simulink model "lab1"  (R2022a)
settings: Solver=FixedStepAuto  StartTime=0.0  StopTime=1e6  RelTol=1e-3
InitFcn:
  | lab1
settings Model: Creator=Natriya  LastModifiedBy=Natriya

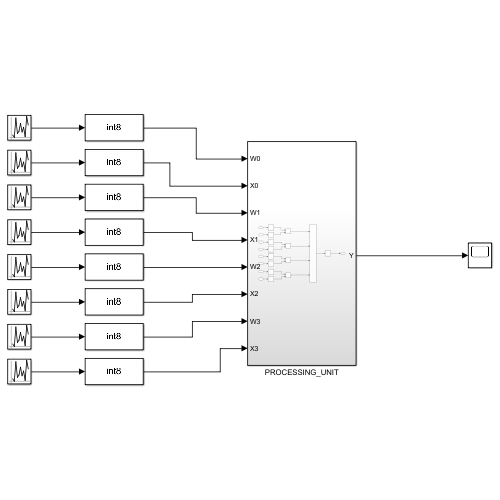
[thumbnail: Simulink's stored preview of the top-level diagram]
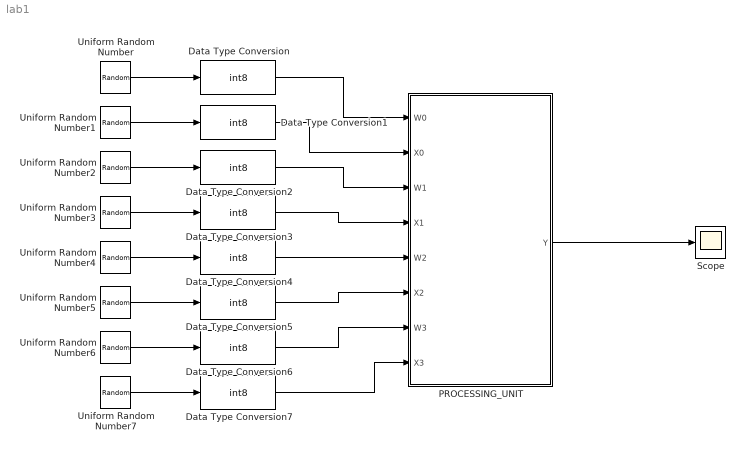
== system lab1 ==
  Data Type Conversion{,1..7} (8 alike) : DataTypeConversion  OutDataTypeStr=int8  SaturateOnIntegerOverflow=off  RndMeth=Floor  LockScale=on
  PROCESSING_UNIT : Subsystem
  Scope : Scope
  Uniform Random Number : UniformRandomNumber  Minimum=0  Maximum=2^8-1  Seed=8  SampleTime=1
  Uniform Random Number1 : UniformRandomNumber  Minimum=0  Maximum=2^8-1  Seed=9  SampleTime=1
  Uniform Random Number2 : UniformRandomNumber  Minimum=0  Maximum=2^8-1  Seed=10  SampleTime=1
  Uniform Random Number3 : UniformRandomNumber  Minimum=0  Maximum=2^8-1  Seed=11  SampleTime=1
  Uniform Random Number4 : UniformRandomNumber  Minimum=0  Maximum=2^8-1  Seed=12  SampleTime=1
  Uniform Random Number5 : UniformRandomNumber  Minimum=0  Maximum=2^8-1  Seed=13  SampleTime=1
  Uniform Random Number6 : UniformRandomNumber  Minimum=0  Maximum=2^8-1  Seed=14  SampleTime=1
  Uniform Random Number7 : UniformRandomNumber  Minimum=0  Maximum=2^8-1  Seed=15  SampleTime=1
  wires:
  Data Type Conversion/1 -> PROCESSING_UNIT/1(W0)
  Data Type Conversion1/1 -> PROCESSING_UNIT/2(X0)
  Data Type Conversion2/1 -> PROCESSING_UNIT/3(W1)
  Data Type Conversion3/1 -> PROCESSING_UNIT/4(X1)
  Data Type Conversion4/1 -> PROCESSING_UNIT/5(W2)
  Data Type Conversion5/1 -> PROCESSING_UNIT/6(X2)
  Data Type Conversion6/1 -> PROCESSING_UNIT/7(W3)
  Data Type Conversion7/1 -> PROCESSING_UNIT/8(X3)
  Uniform Random Number7/1 -> Data Type Conversion7/1
  Uniform Random Number6/1 -> Data Type Conversion6/1
  Uniform Random Number5/1 -> Data Type Conversion5/1
  Uniform Random Number4/1 -> Data Type Conversion4/1
  Uniform Random Number3/1 -> Data Type Conversion3/1
  Uniform Random Number2/1 -> Data Type Conversion2/1
  Uniform Random Number1/1 -> Data Type Conversion1/1
  Uniform Random Number/1 -> Data Type Conversion/1
  PROCESSING_UNIT/1(Y) -> Scope/1

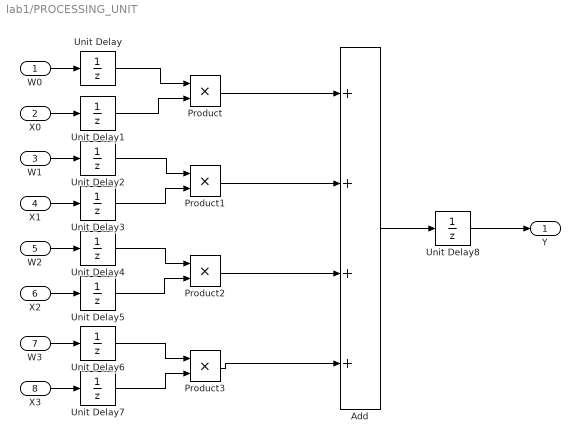
== system lab1/PROCESSING_UNIT ==
  W0 : Inport  OutDataTypeStr=int8  LockScale=on
  X0 : Inport  Port=2  OutDataTypeStr=int8  LockScale=on
  W1 : Inport  Port=3  OutDataTypeStr=int8  LockScale=on
  X1 : Inport  Port=4  OutDataTypeStr=int8  LockScale=on
  W2 : Inport  Port=5  OutDataTypeStr=int8  LockScale=on
  X2 : Inport  Port=6  OutDataTypeStr=int8  LockScale=on
  W3 : Inport  Port=7  OutDataTypeStr=int8  LockScale=on
  X3 : Inport  Port=8  OutDataTypeStr=int8  LockScale=on
  Add : Sum  Inputs=++++  OutDataTypeStr=int16
  Product : Product  OutDataTypeStr=uint16
  Product1 : Product  OutDataTypeStr=int16
  Product2 : Product  OutDataTypeStr=int16
  Product3 : Product  OutDataTypeStr=int16
  Unit Delay{,1..8} (9 alike) : UnitDelay  SampleTime=-1  HasFrameUpgradeWarning=on
  Y : Outport  OutDataTypeStr=int16  LockScale=on
  wires:
  W0/1 -> Unit Delay/1
  X0/1 -> Unit Delay1/1
  W1/1 -> Unit Delay2/1
  X1/1 -> Unit Delay3/1
  W2/1 -> Unit Delay4/1
  X2/1 -> Unit Delay5/1
  W3/1 -> Unit Delay6/1
  X3/1 -> Unit Delay7/1
  Product/1 -> Add/1
  Product1/1 -> Add/2
  Product2/1 -> Add/3
  Product3/1 -> Add/4
  Add/1 -> Unit Delay8/1
  Unit Delay/1 -> Product/1
  Unit Delay1/1 -> Product/2
  Unit Delay2/1 -> Product1/1
  Unit Delay3/1 -> Product1/2
  Unit Delay4/1 -> Product2/1
  Unit Delay5/1 -> Product2/2
  Unit Delay6/1 -> Product3/1
  Unit Delay7/1 -> Product3/2
  Unit Delay8/1 -> Y/1
